simulink model "SensorFusionCompare"  (R2024b)
settings: Solver=FixedStepAuto  StartTime=0.0  StopTime=inf  RelTol=1e-3  EnableMultiTasking=on
values from neighbouring files (symbols this model uses):
  A_kalman = [1 delta_t ... (first row only)    [AttitudePlayground_Vars.m]    (also in ControlSystem_Vars.m)
  acc_sigma = 0.2 * calc_sigma(acc_pp)    [AttitudePlayground_Vars.m]    (also in ControlSystem_Vars.m)
  amfitrack_time = 1    [ControlSystem_Vars.m]
  C_kalman = eye(2)    [AttitudePlayground_Vars.m]    (also in ControlSystem_Vars.m)
  delta_t = 0.01    [AttitudePlayground_Vars.m]    (also in ControlSystem_Vars.m; ParameterIdentification.m = t2 - t1)
  gyro_sigma_3d = [1*gyro_sigma, 1*gyro_sigma, gyro_sigma]    [AttitudePlayground_Vars.m]    (also in ControlSystem_Vars.m)
  inbuilt_reset_time = amfitrack_time + 1    (= 2)    [ControlSystem_Vars.m]
  P_0 = eye(4)    [AttitudePlayground_Vars.m]    (also in ControlSystem_Vars.m)
  q_sigma = 0.001    [AttitudePlayground_Vars.m]    (also in ControlSystem_Vars.m)
  R_kalman = diag([(calc_sigma(0.8))^2, (0.07)^2])    [AttitudePlayground_Vars.m]    (also in ControlSystem_Vars.m)
undefined symbols (not defined in the file or in its folder): Discrete, Time
libraries: simulink_extras x8, dspsigops x2, ctrlSharedLib x1, bbblueSensorLib x1, sharedutil x1, bbblueCommlib x1
settings Model: ExtModeTrigDuration=100  Creator=Henrik  LastModifiedBy=Henrik
settings SolverCC: PositivePriorityOrder=on
settings OptimizationCC: DefaultParameterBehavior=Inlined  EnhancedBackFolding=on  PassReuseOutputArgsAs=Individual arguments  ZeroExternalMemoryAtStartup=off  ZeroInternalMemoryAtStartup=off  MaxStackSize=64  OptimizeBlockOrder=speed  DifferentSizesBufferReuse=on  OptimizationCustomize=off  EfficientTunableParamExpr=on
settings DebuggingCC: ParameterTunabilityLossMsg=error
settings HardwareCC: ProdBitPerPointer=32  ProdBitPerSizeT=32  ProdBitPerPtrDiffT=32  ProdLargestAtomicInteger=Long  ProdLargestAtomicFloat=Double  ProdWordSize=32  ProdHWDeviceType=ARM Compatible->ARM Cortex-A (32-bit)  UseEmbeddedCoderFeatures=off
settings SFSimCC: MATLABDynamicMemAlloc=off
settings RTWCC: Description=Embedded Coder  SystemTargetFile=ert.tlc  HardwareBoard=BeagleBone Blue  TLCOptions="-aInlineSetEventsForThisBaseRateFcn=TLC_FALSE -aSuppressMultiTaskScheduler=TLC_FALSE  -aRateBasedStepFcn=0"  TemplateMakefile=ert_default_tmf  Toolchain=GNU GCC BeagleBone Blue
settings CodeAppCC: ForceParamTrailComments=on  IgnoreCustomStorageClasses=off  OperatorAnnotations=on  SimulinkDataObjDesc=on  SFDataObjDesc=on  InsertBlockDesc=on
settings ERTTargetCC: SupportNonInlinedSFcns=on  SupportVariableSizeSignals=on

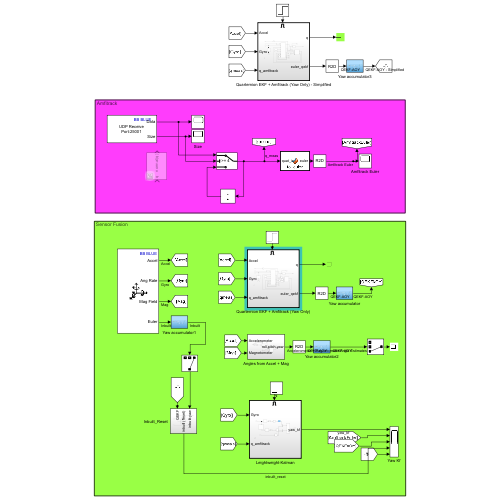
[thumbnail: Simulink's stored preview of the top-level diagram]
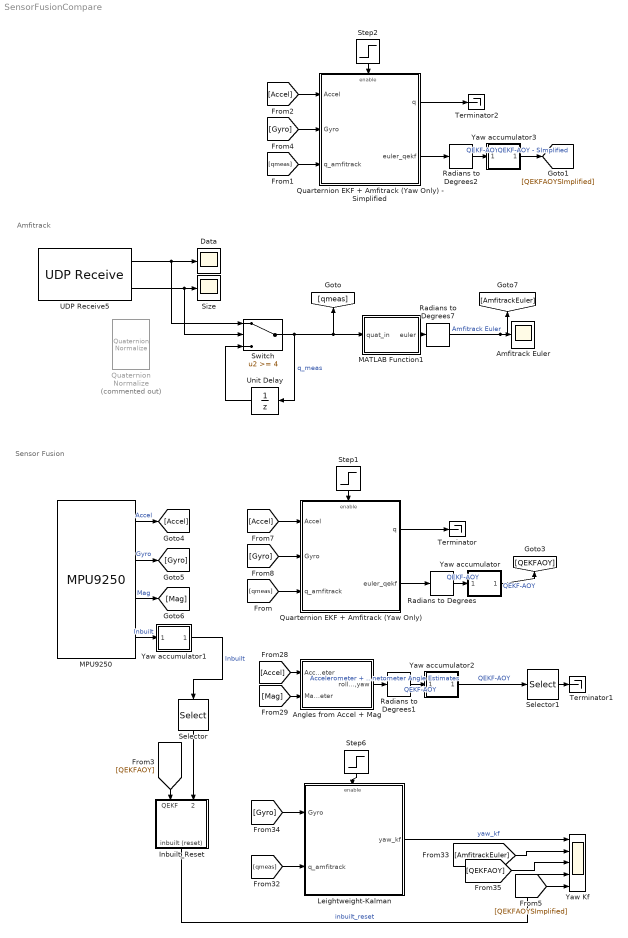
== system SensorFusionCompare ==
  note: Sensor Fusion
  note: Amfitrack
  Amfitrack Euler : Scope
  Angles from Accel + Mag : Subsystem
  Data : Scope
  Inbuilt_Reset : Subsystem
  Leightweight-Kalman : Subsystem
  MATLAB Function1 : MATLAB Function  TreatAsAtomicUnit=on
  MPU9250 : bbblueSensorLib/MPU9250  OperationMode=DMP  Accel=on  AngularRate=on  Ak8963Field=on  EulerAngles=on  Quat=off  AccelRange=2G  Acceldlpf=1  GyroRange=250 dps  Gyrodlpf=1  DmpOdr=200 Hz  SampleTime=delta_t
  Quarternion EKF + Amfitrack (Yaw Only) : Subsystem
  Quarternion EKF + Amfitrack (Yaw Only) - Simplified : Subsystem
  Quaternion Normalize : sharedutil/Quaternion Normalize  Commented=on  aMode=aMode
  Radians to Degrees{,1..2,7} (4 alike) : simulink_extras/Transformations/Radians to Degrees
  Selector : Selector  InputPortWidth=3  IndexOptions=Index vector (dialog)  Indices=[3]  OutputSizes=1
  Selector1 : Selector  InputPortWidth=3  IndexOptions=Index vector (dialog)  Indices=[3]  OutputSizes=1
  Size : Scope
  Step1 : Step  Time=amfitrack_time  SampleTime=delta_t
  Step2 : Step  Time=amfitrack_time  SampleTime=delta_t
  Step6 : Step  Time=amfitrack_time  SampleTime=delta_t
  Switch : Switch  Threshold=4  SaturateOnIntegerOverflow=off  InputSameDT=off
  Terminator : Terminator
  Terminator1 : Terminator
  Terminator2 : Terminator
  UDP Receive5 : bbblueCommlib/UDP Receive  localURL='0.0.0.0'  localPort=25001  remoteURL='0.0.0.0'  remotePort=-1  recvBufferSize=8192  signalDatatype=double  dims=4  isVarSize=off  showBlockingTime=off  blockingTime=0  sampletime=delta_t  blockPlatform=BB BLUE
  Unit Delay : UnitDelay  InitialCondition=[1,0,0,0]'  SampleTime=-1  HasFrameUpgradeWarning=on
  Yaw Kf : Scope  NumInputPorts=5
  Yaw accumulator : Subsystem
  Yaw accumulator1 : Subsystem
  Yaw accumulator2 : Subsystem
  Yaw accumulator3 : Subsystem
  wires:
  MPU9250/1 -> [Accel]  "Accel"
  [Accel] -> Quarternion EKF + Amfitrack (Yaw Only)/1(Accel)
  Radians to Degrees/1 -> Yaw accumulator/1(yaw)  "QEKF-AOY"
  Step1/1 -> Quarternion EKF + Amfitrack (Yaw Only)/Enable
  [Gyro] -> Quarternion EKF + Amfitrack (Yaw Only)/2(Gyro)
  MPU9250/4 -> Yaw accumulator1/1(yaw)  "Inbuilt"
  Angles from Accel + Mag/1(roll,pitch,yaw) -> Radians to Degrees1/1  "Accelerometer + Magnetometer Angle Estimates"
  Quarternion EKF + Amfitrack (Yaw Only)/1(q) -> Terminator/1
  [Accel] -> Angles from Accel + Mag/1(Accelerometer)
  Yaw accumulator2/1(yaw_acc) -> Selector1/1  "QEKF-AOY"
  MPU9250/2 -> [Gyro]  "Gyro"
  Yaw accumulator/1(yaw_acc) -> [QEKFAOY]  "QEKF-AOY"
  Quarternion EKF + Amfitrack (Yaw Only)/2(euler_qekf) -> Radians to Degrees/1
  [qmeas] -> Quarternion EKF + Amfitrack (Yaw Only)/3(q_amfitrack)
  MPU9250/3 -> [Mag]  "Mag"
  Radians to Degrees1/1 -> Yaw accumulator2/1(yaw)  "QEKF-AOY"
  Yaw accumulator1/1(yaw_acc) -> Selector/1  "Inbuilt"
  [Mag] -> Angles from Accel + Mag/2(Magnetometer)
  [AmfitrackEuler] -> Yaw Kf/2
  [Gyro] -> Leightweight-Kalman/1(Gyro)
  Leightweight-Kalman/1(yaw_kf) -> Yaw Kf/1  "yaw_kf"
  [QEKFAOY] -> Yaw Kf/3
  [qmeas] -> Leightweight-Kalman/2(q_amfitrack)
  Step6/1 -> Leightweight-Kalman/Enable
  UDP Receive5/1 -> Switch/1, Data/1
  Switch/1 -> MATLAB Function1/1(quat_in), [qmeas], Unit Delay/1  "q_meas"
  Radians to Degrees7/1 -> Amfitrack Euler/1, [AmfitrackEuler]  "Amfitrack Euler"
  MATLAB Function1/1(euler) -> Radians to Degrees7/1
  Unit Delay/1 -> Switch/3
  UDP Receive5/2 -> Switch/2, Size/1
  [QEKFAOY] -> Inbuilt_Reset/1(QEKF)
  Selector/1 -> Inbuilt_Reset/2(inbuilt-yaw)
  Inbuilt_Reset/1(inbuilt (reset)) -> Yaw Kf/4  "inbuilt_reset"
  Selector1/1 -> Terminator1/1
  [qmeas] -> Quarternion EKF + Amfitrack (Yaw Only) - Simplified/3(q_amfitrack)
  Quarternion EKF + Amfitrack (Yaw Only) - Simplified/2(euler_qekf) -> Radians to Degrees2/1
  Quarternion EKF + Amfitrack (Yaw Only) - Simplified/1(q) -> Terminator2/1
  [Gyro] -> Quarternion EKF + Amfitrack (Yaw Only) - Simplified/2(Gyro)
  Step2/1 -> Quarternion EKF + Amfitrack (Yaw Only) - Simplified/Enable
  Radians to Degrees2/1 -> Yaw accumulator3/1(yaw)  "QEKF-AOY"
  [Accel] -> Quarternion EKF + Amfitrack (Yaw Only) - Simplified/1(Accel)
  Yaw accumulator3/1(yaw_acc) -> [QEKFAOYSImplified]  "QEKF-AOY - SImplified"
  [QEKFAOYSImplified] -> Yaw Kf/5

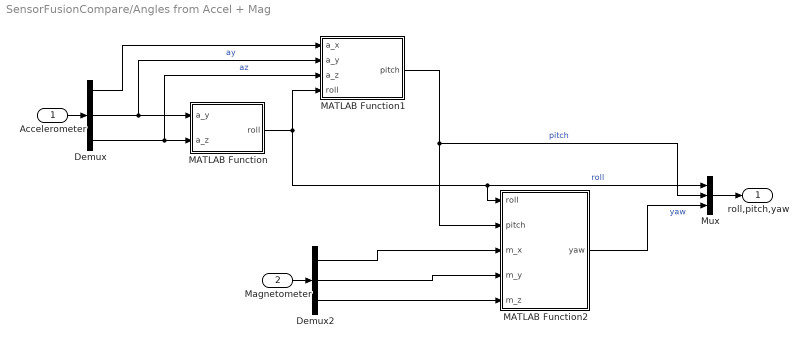
== system SensorFusionCompare/Angles from Accel + Mag ==
  Accelerometer : Inport
  Magnetometer : Inport  Port=2
  Demux : Demux  Outputs=3
  Demux2 : Demux  Outputs=3
  MATLAB Function : MATLAB Function  TreatAsAtomicUnit=on
  MATLAB Function1 : MATLAB Function  TreatAsAtomicUnit=on
  MATLAB Function2 : MATLAB Function  TreatAsAtomicUnit=on
  Mux : Mux  Inputs=3
  roll,pitch,yaw : Outport
  wires:
  Accelerometer/1 -> Demux/1
  Demux/1 -> MATLAB Function1/1(a_x)
  Demux/3 -> MATLAB Function1/3(a_z), MATLAB Function/2(a_z)  "az"
  Demux/2 -> MATLAB Function1/2(a_y), MATLAB Function/1(a_y)  "ay"
  Magnetometer/1 -> Demux2/1
  MATLAB Function/1(roll) -> MATLAB Function1/4(roll), Mux/1, MATLAB Function2/1(roll)  "roll"
  MATLAB Function1/1(pitch) -> Mux/2, MATLAB Function2/2(pitch)  "pitch"
  Demux2/1 -> MATLAB Function2/3(m_x)
  Demux2/2 -> MATLAB Function2/4(m_y)
  Demux2/3 -> MATLAB Function2/5(m_z)
  Mux/1 -> roll,pitch,yaw/1
  MATLAB Function2/1(yaw) -> Mux/3  "yaw"

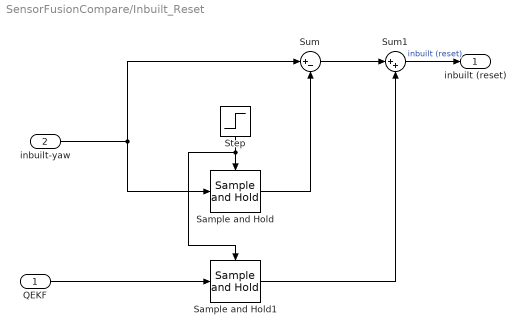
== system SensorFusionCompare/Inbuilt_Reset ==
  QEKF : Inport
  inbuilt-yaw : Inport  Port=2
  Sample and Hold : dspsigops/Sample and Hold  trig=Rising edge  initCond=0  latchinput=off
  Sample and Hold1 : dspsigops/Sample and Hold  trig=Rising edge  initCond=0  latchinput=off
  Step : Step  Time=inbuilt_reset_time  SampleTime=0
  Sum : Sum  Inputs=|+-
  Sum1 : Sum  Inputs=|++
  inbuilt (reset) : Outport
  wires:
  Step/1 -> Sample and Hold1/Trigger, Sample and Hold/Trigger
  Sum/1 -> Sum1/1
  Sample and Hold/1 -> Sum/2
  inbuilt-yaw/1 -> Sum/1, Sample and Hold/1
  Sample and Hold1/1 -> Sum1/2
  Sum1/1 -> inbuilt (reset)/1  "inbuilt (reset)"
  QEKF/1 -> Sample and Hold1/1

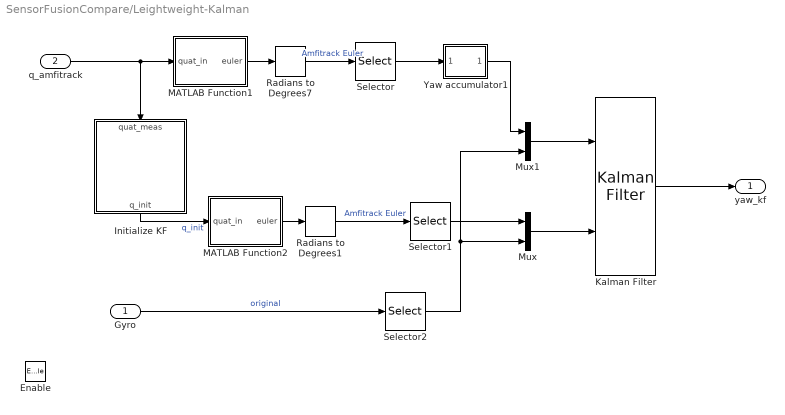
== system SensorFusionCompare/Leightweight-Kalman ==
  Gyro : Inport
  q_amfitrack : Inport  Port=2
  Enable : EnablePort
  Initialize KF : MATLAB Function  TreatAsAtomicUnit=on
  Kalman Filter : ctrlSharedLib/Kalman Filter  TimeDomain=Discrete-Time  UseCurrentEstimator=on  ModelSource=Individual A, B, C, D matrices  ModelSourceVariable=ss(0.95,1,1,0,1)  A=A_kalman  B=1  C=C_kalman  D=0  NumberOfStates=1  NumberOfInputs=1  NumberOfOutputs=1  InitialEstimateSource=Input port  X0=0  P0=10  UseK=off  UseGH=off  NumberOfProcessNoiseInputs=1  G=1  TimeInvariantG=on  H=0  TimeInvariantH=on  Q=Q_kalman  TimeInvariantQ=on  R=R_kalman  TimeInvariantR=on  N=0  TimeInvariantN=on  AddInputPort=off  AddEnablePort=off  OutputEstimatedY=off  OutputP=off  Ts=-1
  MATLAB Function1 : MATLAB Function  TreatAsAtomicUnit=on
  MATLAB Function2 : MATLAB Function  TreatAsAtomicUnit=on
  Mux : Mux  Inputs=2
  Mux1 : Mux  Inputs=2
  Radians to Degrees1 : simulink_extras/Transformations/Radians to Degrees
  Radians to Degrees7 : simulink_extras/Transformations/Radians to Degrees
  Selector : Selector  InputPortWidth=3  IndexOptions=Index vector (dialog)  Indices=[3]  OutputSizes=1
  Selector1 : Selector  InputPortWidth=3  IndexOptions=Index vector (dialog)  Indices=[3]  OutputSizes=1
  Selector2 : Selector  InputPortWidth=3  IndexOptions=Index vector (dialog)  Indices=[3]  OutputSizes=1
  Yaw accumulator1 : Subsystem
  yaw_kf : Outport
  wires:
  Gyro/1 -> Selector2/1  "original"
  q_amfitrack/1 -> MATLAB Function1/1(quat_in), Initialize KF/1(quat_meas)
  Initialize KF/1(q_init) -> MATLAB Function2/1(quat_in)  "q_init"
  Radians to Degrees7/1 -> Selector/1  "Amfitrack Euler"
  MATLAB Function1/1(euler) -> Radians to Degrees7/1
  MATLAB Function2/1(euler) -> Radians to Degrees1/1
  Radians to Degrees1/1 -> Selector1/1  "Amfitrack Euler"
  Selector1/1 -> Mux/1
  Mux/1 -> Kalman Filter/2
  Kalman Filter/1 -> yaw_kf/1
  Selector/1 -> Yaw accumulator1/1(yaw)
  Mux1/1 -> Kalman Filter/1
  Yaw accumulator1/1(yaw_acc) -> Mux1/1
  Selector2/1 -> Mux1/2, Mux/2

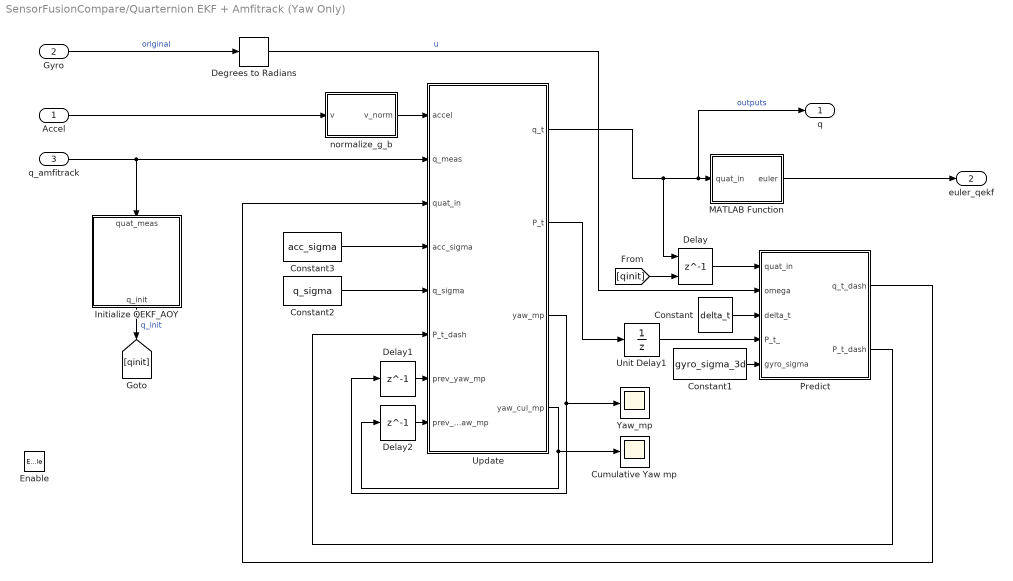
== system SensorFusionCompare/Quarternion EKF + Amfitrack (Yaw Only) ==
  Accel : Inport
  Gyro : Inport  Port=2
  q_amfitrack : Inport  Port=3
  Enable : EnablePort
  Constant : Constant  Value=delta_t
  Constant1 : Constant  Value=gyro_sigma_3d
  Constant2 : Constant  Value=q_sigma
  Constant3 : Constant  Value=acc_sigma
  Cumulative Yaw mp : Scope
  Degrees to Radians : simulink_extras/Transformations/Degrees to Radians
  Delay : Delay  DelayLength=1  InitialConditionSource=Input port  InitialCondition=[1,0,0,0]  SampleTime=delta_t
      settings: InputPortMap=u0,p4
  Delay1 : Delay  DelayLength=1  InitialCondition=[0,0]  SampleTime=delta_t
  Delay2 : Delay  DelayLength=1  InitialCondition=[0,0]  SampleTime=delta_t
  Initialize QEKF_AOY : MATLAB Function  TreatAsAtomicUnit=on
  MATLAB Function : MATLAB Function  TreatAsAtomicUnit=on
  Predict : MATLAB Function  TreatAsAtomicUnit=on
  Unit Delay1 : UnitDelay  InitialCondition=P_0  SampleTime=delta_t  HasFrameUpgradeWarning=on
  Update : MATLAB Function  TreatAsAtomicUnit=on  SystemSampleTime=delta_t
  Yaw_mp : Scope
  normalize_g_b : MATLAB Function  TreatAsAtomicUnit=on
  q : Outport
  euler_qekf : Outport  Port=2
  wires:
  Update/1(q_t) -> Delay/1, q/1, MATLAB Function/1(quat_in)  "outputs"
  Accel/1 -> normalize_g_b/1(v)
  Constant/1 -> Predict/3(delta_t)
  Unit Delay1/1 -> Predict/4(P_t_)
  Update/2(P_t) -> Unit Delay1/1
  Predict/1(q_t_dash) -> Update/3(quat_in)
  normalize_g_b/1(v_norm) -> Update/1(accel)
  Constant3/1 -> Update/4(acc_sigma)
  Delay/1 -> Predict/1(quat_in)
  Predict/2(P_t_dash) -> Update/6(P_t_dash)
  MATLAB Function/1(euler) -> euler_qekf/1
  Degrees to Radians/1 -> Predict/2(omega)  "u"
  Gyro/1 -> Degrees to Radians/1  "original"
  Constant1/1 -> Predict/5(gyro_sigma)
  q_amfitrack/1 -> Update/2(q_meas), Initialize QEKF_AOY/1(quat_meas)
  Constant2/1 -> Update/5(q_sigma)
  Delay1/1 -> Update/7(prev_yaw_mp)
  Delay2/1 -> Update/8(prev_cul_yaw_mp)
  Update/3(yaw_mp) -> Delay1/1, Yaw_mp/1
  Update/4(yaw_cul_mp) -> Delay2/1, Cumulative Yaw mp/1
  Initialize QEKF_AOY/1(q_init) -> [qinit]  "q_init"
  [qinit] -> Delay/2

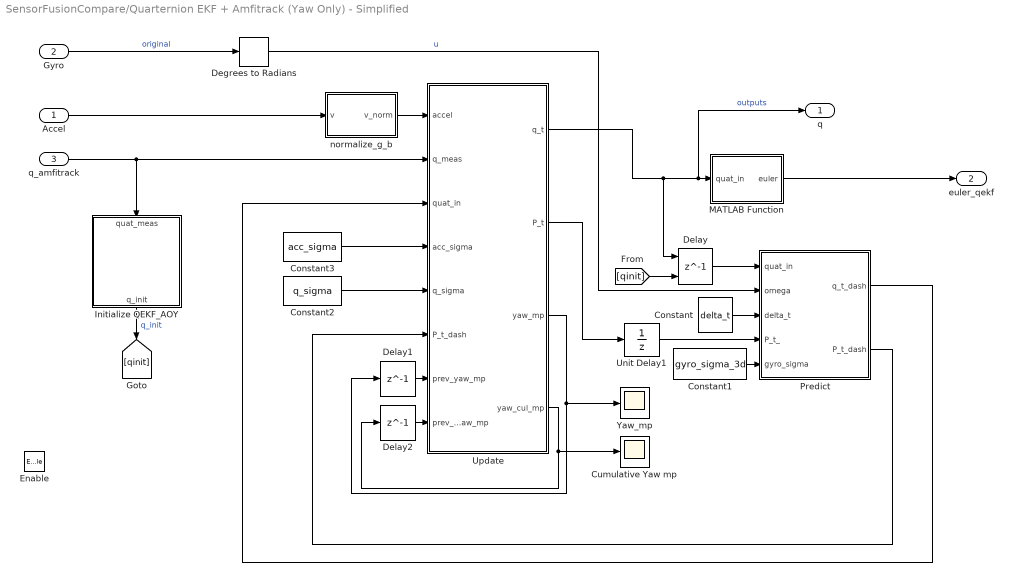
== system SensorFusionCompare/Quarternion EKF + Amfitrack (Yaw Only) - Simplified ==
  Accel : Inport
  Gyro : Inport  Port=2
  q_amfitrack : Inport  Port=3
  Enable : EnablePort
  Constant : Constant  Value=delta_t
  Constant1 : Constant  Value=gyro_sigma_3d
  Constant2 : Constant  Value=q_sigma
  Constant3 : Constant  Value=acc_sigma
  Cumulative Yaw mp : Scope
  Degrees to Radians : simulink_extras/Transformations/Degrees to Radians
  Delay : Delay  DelayLength=1  InitialConditionSource=Input port  InitialCondition=[1,0,0,0]  SampleTime=delta_t
      settings: InputPortMap=u0,p4
  Delay1 : Delay  DelayLength=1  InitialCondition=[0,0]  SampleTime=delta_t
  Delay2 : Delay  DelayLength=1  InitialCondition=[0,0]  SampleTime=delta_t
  Initialize QEKF_AOY : MATLAB Function  TreatAsAtomicUnit=on
  MATLAB Function : MATLAB Function  TreatAsAtomicUnit=on
  Predict : MATLAB Function  TreatAsAtomicUnit=on
  Unit Delay1 : UnitDelay  InitialCondition=P_0  SampleTime=delta_t  HasFrameUpgradeWarning=on
  Update : MATLAB Function  TreatAsAtomicUnit=on  SystemSampleTime=delta_t
  Yaw_mp : Scope
  normalize_g_b : MATLAB Function  TreatAsAtomicUnit=on
  q : Outport
  euler_qekf : Outport  Port=2
  wires:
  [qinit] -> Delay/2
  Initialize QEKF_AOY/1(q_init) -> [qinit]  "q_init"
  Update/4(yaw_cul_mp) -> Cumulative Yaw mp/1, Delay2/1
  Update/3(yaw_mp) -> Yaw_mp/1, Delay1/1
  Delay2/1 -> Update/8(prev_cul_yaw_mp)
  Delay1/1 -> Update/7(prev_yaw_mp)
  Constant2/1 -> Update/5(q_sigma)
  q_amfitrack/1 -> Initialize QEKF_AOY/1(quat_meas), Update/2(q_meas)
  Constant1/1 -> Predict/5(gyro_sigma)
  Gyro/1 -> Degrees to Radians/1  "original"
  Degrees to Radians/1 -> Predict/2(omega)  "u"
  MATLAB Function/1(euler) -> euler_qekf/1
  Predict/2(P_t_dash) -> Update/6(P_t_dash)
  Delay/1 -> Predict/1(quat_in)
  Constant3/1 -> Update/4(acc_sigma)
  normalize_g_b/1(v_norm) -> Update/1(accel)
  Predict/1(q_t_dash) -> Update/3(quat_in)
  Update/2(P_t) -> Unit Delay1/1
  Unit Delay1/1 -> Predict/4(P_t_)
  Constant/1 -> Predict/3(delta_t)
  Accel/1 -> normalize_g_b/1(v)
  Update/1(q_t) -> MATLAB Function/1(quat_in), q/1, Delay/1  "outputs"

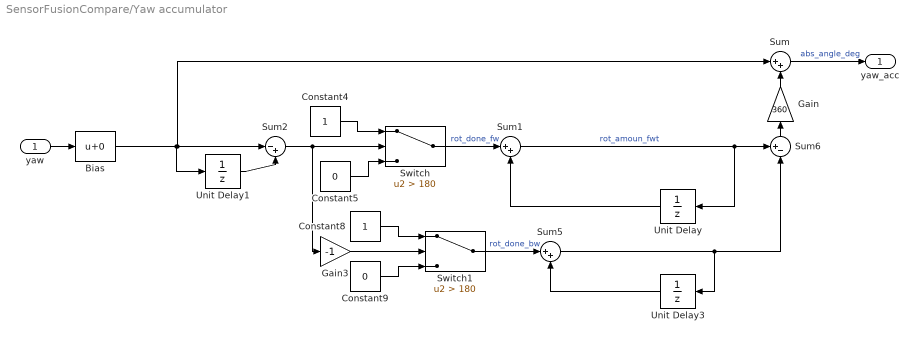
== system SensorFusionCompare/Yaw accumulator ==
  yaw : Inport
  Bias : Bias  SaturateOnIntegerOverflow=off
  Constant4 : Constant
  Constant5 : Constant  Value=0
  Constant8 : Constant
  Constant9 : Constant  Value=0
  Gain : Gain  Gain=360
  Gain3 : Gain  Gain=-1
  Sum : Sum  Inputs=|++
  Sum1 : Sum  Inputs=|++
  Sum2 : Sum  Inputs=|-+
  Sum5 : Sum  Inputs=|++
  Sum6 : Sum  Inputs=+-|
  Switch : Switch  Criteria=u2 > Threshold  Threshold=180  SaturateOnIntegerOverflow=off  InputSameDT=off
  Switch1 : Switch  Criteria=u2 > Threshold  Threshold=180  SaturateOnIntegerOverflow=off  InputSameDT=off
  Unit Delay : UnitDelay  SampleTime=-1  HasFrameUpgradeWarning=on
  Unit Delay1 : UnitDelay  SampleTime=-1  HasFrameUpgradeWarning=on
  Unit Delay3 : UnitDelay  SampleTime=-1  HasFrameUpgradeWarning=on
  yaw_acc : Outport
  wires:
  Sum1/1 -> Unit Delay/1, Sum6/1  "rot_amoun_fwt"
  Constant5/1 -> Switch/3
  Constant8/1 -> Switch1/1
  Sum5/1 -> Unit Delay3/1, Sum6/2
  Sum6/1 -> Gain/1
  Unit Delay/1 -> Sum1/2
  Constant4/1 -> Switch/1
  yaw/1 -> Bias/1
  Unit Delay3/1 -> Sum5/2
  Switch/1 -> Sum1/1  "rot_done_fw"
  Sum2/1 -> Gain3/1, Switch/2
  Gain3/1 -> Switch1/2
  Unit Delay1/1 -> Sum2/2
  Sum/1 -> yaw_acc/1  "abs_angle_deg"
  Switch1/1 -> Sum5/1  "rot_done_bw"
  Constant9/1 -> Switch1/3
  Gain/1 -> Sum/2
  Bias/1 -> Unit Delay1/1, Sum/1, Sum2/1

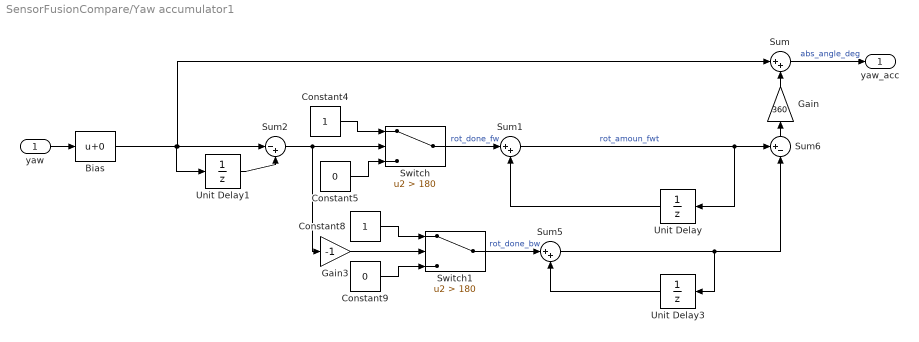
== system SensorFusionCompare/Yaw accumulator1 ==
  yaw : Inport
  Bias : Bias  SaturateOnIntegerOverflow=off
  Constant4 : Constant
  Constant5 : Constant  Value=0
  Constant8 : Constant
  Constant9 : Constant  Value=0
  Gain : Gain  Gain=360
  Gain3 : Gain  Gain=-1
  Sum : Sum  Inputs=|++
  Sum1 : Sum  Inputs=|++
  Sum2 : Sum  Inputs=|-+
  Sum5 : Sum  Inputs=|++
  Sum6 : Sum  Inputs=+-|
  Switch : Switch  Criteria=u2 > Threshold  Threshold=180  SaturateOnIntegerOverflow=off  InputSameDT=off
  Switch1 : Switch  Criteria=u2 > Threshold  Threshold=180  SaturateOnIntegerOverflow=off  InputSameDT=off
  Unit Delay : UnitDelay  SampleTime=-1  HasFrameUpgradeWarning=on
  Unit Delay1 : UnitDelay  SampleTime=-1  HasFrameUpgradeWarning=on
  Unit Delay3 : UnitDelay  SampleTime=-1  HasFrameUpgradeWarning=on
  yaw_acc : Outport
  wires:
  Sum1/1 -> Unit Delay/1, Sum6/1  "rot_amoun_fwt"
  Constant5/1 -> Switch/3
  Constant8/1 -> Switch1/1
  Sum5/1 -> Unit Delay3/1, Sum6/2
  Sum6/1 -> Gain/1
  Unit Delay/1 -> Sum1/2
  Constant4/1 -> Switch/1
  yaw/1 -> Bias/1
  Unit Delay3/1 -> Sum5/2
  Switch/1 -> Sum1/1  "rot_done_fw"
  Sum2/1 -> Gain3/1, Switch/2
  Gain3/1 -> Switch1/2
  Unit Delay1/1 -> Sum2/2
  Sum/1 -> yaw_acc/1  "abs_angle_deg"
  Switch1/1 -> Sum5/1  "rot_done_bw"
  Constant9/1 -> Switch1/3
  Gain/1 -> Sum/2
  Bias/1 -> Unit Delay1/1, Sum/1, Sum2/1

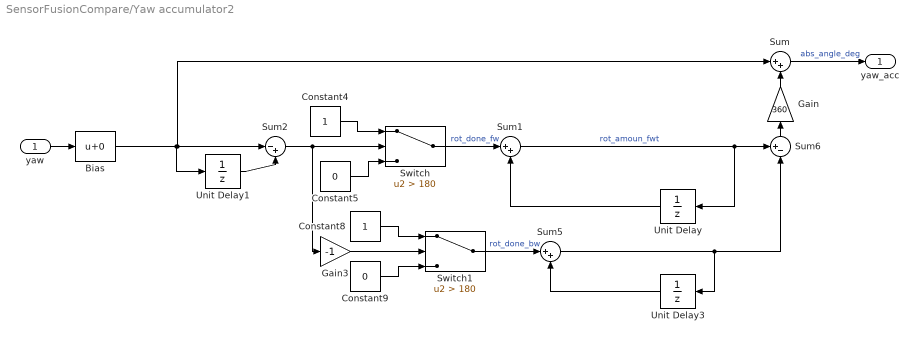
== system SensorFusionCompare/Yaw accumulator2 ==
  yaw : Inport
  Bias : Bias  SaturateOnIntegerOverflow=off
  Constant4 : Constant
  Constant5 : Constant  Value=0
  Constant8 : Constant
  Constant9 : Constant  Value=0
  Gain : Gain  Gain=360
  Gain3 : Gain  Gain=-1
  Sum : Sum  Inputs=|++
  Sum1 : Sum  Inputs=|++
  Sum2 : Sum  Inputs=|-+
  Sum5 : Sum  Inputs=|++
  Sum6 : Sum  Inputs=+-|
  Switch : Switch  Criteria=u2 > Threshold  Threshold=180  SaturateOnIntegerOverflow=off  InputSameDT=off
  Switch1 : Switch  Criteria=u2 > Threshold  Threshold=180  SaturateOnIntegerOverflow=off  InputSameDT=off
  Unit Delay : UnitDelay  SampleTime=-1  HasFrameUpgradeWarning=on
  Unit Delay1 : UnitDelay  SampleTime=-1  HasFrameUpgradeWarning=on
  Unit Delay3 : UnitDelay  SampleTime=-1  HasFrameUpgradeWarning=on
  yaw_acc : Outport
  wires:
  Bias/1 -> Sum2/1, Sum/1, Unit Delay1/1
  Gain/1 -> Sum/2
  Constant9/1 -> Switch1/3
  Switch1/1 -> Sum5/1  "rot_done_bw"
  Sum/1 -> yaw_acc/1  "abs_angle_deg"
  Unit Delay1/1 -> Sum2/2
  Gain3/1 -> Switch1/2
  Sum2/1 -> Switch/2, Gain3/1
  Switch/1 -> Sum1/1  "rot_done_fw"
  Unit Delay3/1 -> Sum5/2
  yaw/1 -> Bias/1
  Constant4/1 -> Switch/1
  Unit Delay/1 -> Sum1/2
  Sum6/1 -> Gain/1
  Sum5/1 -> Sum6/2, Unit Delay3/1
  Constant8/1 -> Switch1/1
  Constant5/1 -> Switch/3
  Sum1/1 -> Sum6/1, Unit Delay/1  "rot_amoun_fwt"

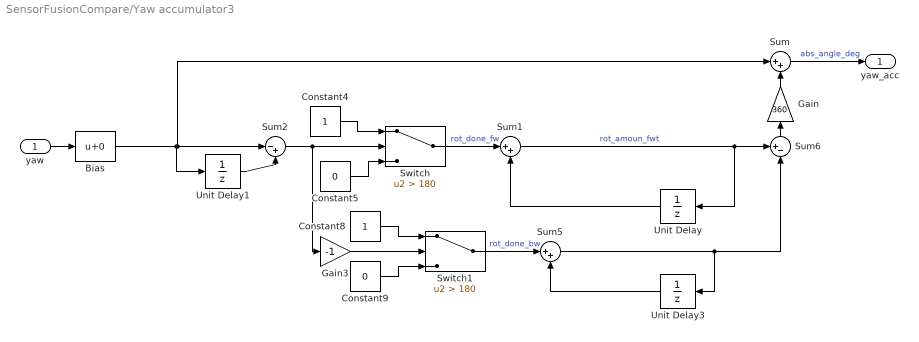
== system SensorFusionCompare/Yaw accumulator3 ==
  yaw : Inport
  Bias : Bias  SaturateOnIntegerOverflow=off
  Constant4 : Constant
  Constant5 : Constant  Value=0
  Constant8 : Constant
  Constant9 : Constant  Value=0
  Gain : Gain  Gain=360
  Gain3 : Gain  Gain=-1
  Sum : Sum  Inputs=|++
  Sum1 : Sum  Inputs=|++
  Sum2 : Sum  Inputs=|-+
  Sum5 : Sum  Inputs=|++
  Sum6 : Sum  Inputs=+-|
  Switch : Switch  Criteria=u2 > Threshold  Threshold=180  SaturateOnIntegerOverflow=off  InputSameDT=off
  Switch1 : Switch  Criteria=u2 > Threshold  Threshold=180  SaturateOnIntegerOverflow=off  InputSameDT=off
  Unit Delay : UnitDelay  SampleTime=-1  HasFrameUpgradeWarning=on
  Unit Delay1 : UnitDelay  SampleTime=-1  HasFrameUpgradeWarning=on
  Unit Delay3 : UnitDelay  SampleTime=-1  HasFrameUpgradeWarning=on
  yaw_acc : Outport
  wires:
  Bias/1 -> Sum2/1, Sum/1, Unit Delay1/1
  Gain/1 -> Sum/2
  Constant9/1 -> Switch1/3
  Switch1/1 -> Sum5/1  "rot_done_bw"
  Sum/1 -> yaw_acc/1  "abs_angle_deg"
  Unit Delay1/1 -> Sum2/2
  Gain3/1 -> Switch1/2
  Sum2/1 -> Switch/2, Gain3/1
  Switch/1 -> Sum1/1  "rot_done_fw"
  Unit Delay3/1 -> Sum5/2
  yaw/1 -> Bias/1
  Constant4/1 -> Switch/1
  Unit Delay/1 -> Sum1/2
  Sum6/1 -> Gain/1
  Sum5/1 -> Sum6/2, Unit Delay3/1
  Constant8/1 -> Switch1/1
  Constant5/1 -> Switch/3
  Sum1/1 -> Sum6/1, Unit Delay/1  "rot_amoun_fwt"

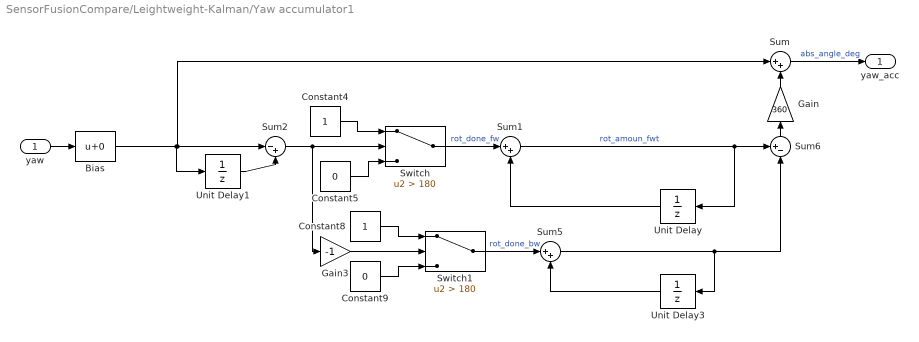
== system SensorFusionCompare/Leightweight-Kalman/Yaw accumulator1 ==
  yaw : Inport
  Bias : Bias  SaturateOnIntegerOverflow=off
  Constant4 : Constant
  Constant5 : Constant  Value=0
  Constant8 : Constant
  Constant9 : Constant  Value=0
  Gain : Gain  Gain=360
  Gain3 : Gain  Gain=-1
  Sum : Sum  Inputs=|++
  Sum1 : Sum  Inputs=|++
  Sum2 : Sum  Inputs=|-+
  Sum5 : Sum  Inputs=|++
  Sum6 : Sum  Inputs=+-|
  Switch : Switch  Criteria=u2 > Threshold  Threshold=180  SaturateOnIntegerOverflow=off  InputSameDT=off
  Switch1 : Switch  Criteria=u2 > Threshold  Threshold=180  SaturateOnIntegerOverflow=off  InputSameDT=off
  Unit Delay : UnitDelay  SampleTime=-1  HasFrameUpgradeWarning=on
  Unit Delay1 : UnitDelay  SampleTime=-1  HasFrameUpgradeWarning=on
  Unit Delay3 : UnitDelay  SampleTime=-1  HasFrameUpgradeWarning=on
  yaw_acc : Outport
  wires:
  Sum1/1 -> Unit Delay/1, Sum6/1  "rot_amoun_fwt"
  Constant5/1 -> Switch/3
  Constant8/1 -> Switch1/1
  Sum5/1 -> Unit Delay3/1, Sum6/2
  Sum6/1 -> Gain/1
  Unit Delay/1 -> Sum1/2
  Constant4/1 -> Switch/1
  yaw/1 -> Bias/1
  Unit Delay3/1 -> Sum5/2
  Switch/1 -> Sum1/1  "rot_done_fw"
  Sum2/1 -> Gain3/1, Switch/2
  Gain3/1 -> Switch1/2
  Unit Delay1/1 -> Sum2/2
  Sum/1 -> yaw_acc/1  "abs_angle_deg"
  Switch1/1 -> Sum5/1  "rot_done_bw"
  Constant9/1 -> Switch1/3
  Gain/1 -> Sum/2
  Bias/1 -> Unit Delay1/1, Sum/1, Sum2/1

== matlab function SensorFusionCompare/Leightweight-Kalman/Initialize KF ==
  data: quat_meas input; q_init output
function q_init = calc_init_q(quat_meas)

q0 = quat_meas(1);
q1 = quat_meas(2);
q2 = quat_meas(3);
q3 = quat_meas(4);


yaw_init_rad = atan2((2 * (q0*q3 + q1*q2)),(1 - 2*(q2^2 + q3^2)));
q_init = [cos(yaw_init_rad/2), 0, 0, sin(yaw_init_rad/2)];

== matlab function SensorFusionCompare/Leightweight-Kalman/MATLAB Function1 ==
  data: quat_in input; euler output
function euler = to_euler(quat_in)

q0 = quat_in(1);
q1 = quat_in(2);
q2 = quat_in(3);
q3 = quat_in(4);

roll = atan((2 * (q0*q1 + q2*q3))/(1 - 2*(q1^2 + q2^2)));
pitch = asin(2 * (q0*q2 - q1*q3));
yaw = atan2((2 * (q0*q3 + q1*q2)),(1 - 2*(q2^2 + q3^2)));

euler = [roll; pitch; yaw];

== matlab function SensorFusionCompare/Leightweight-Kalman/MATLAB Function2 ==
  data: quat_in input; euler output
function euler = to_euler(quat_in)

q0 = quat_in(1);
q1 = quat_in(2);
q2 = quat_in(3);
q3 = quat_in(4);

roll = atan((2 * (q0*q1 + q2*q3))/(1 - 2*(q1^2 + q2^2)));
pitch = asin(2 * (q0*q2 - q1*q3));
yaw = atan2((2 * (q0*q3 + q1*q2)),(1 - 2*(q2^2 + q3^2)));

euler = [roll; pitch; yaw];

== matlab function SensorFusionCompare/MATLAB Function1 ==
  data: quat_in input; euler output
function euler = to_euler(quat_in)

q0 = quat_in(1);
q1 = quat_in(2);
q2 = quat_in(3);
q3 = quat_in(4);

roll = atan((2 * (q0*q1 + q2*q3))/(1 - 2*(q1^2 + q2^2)));
pitch = asin(2 * (q0*q2 - q1*q3));
yaw = atan2((2 * (q0*q3 + q1*q2)),(1 - 2*(q2^2 + q3^2)));

euler = [roll; pitch; yaw];

== matlab function SensorFusionCompare/Quarternion EKF + Amfitrack (Yaw Only)/MATLAB Function ==
  data: quat_in input; euler output
function euler = to_euler(quat_in)

q0 = quat_in(1);
q1 = quat_in(2);
q2 = quat_in(3);
q3 = quat_in(4);

roll = atan((2 * (q0*q1 + q2*q3))/(1 - 2*(q1^2 + q2^2)));
pitch = asin(2 * (q0*q2 - q1*q3));
yaw = atan2((2 * (q0*q3 + q1*q2)),(1 - 2*(q2^2 + q3^2)));

euler = [roll; pitch; yaw];

== matlab function SensorFusionCompare/Quarternion EKF + Amfitrack (Yaw Only)/Predict ==
  data: quat_in input; q_t_dash output; omega input; delta_t input; P_t_dash output; P_t_ input; gyro_sigma input
function [q_t_dash, P_t_dash] = Predict(quat_in, omega, delta_t, P_t_, gyro_sigma)

q0 = quat_in(1);
q1 = quat_in(2);
q2 = quat_in(3);
q3 = quat_in(4);

omega_x = omega(1);
omega_y = omega(2);
omega_z = omega(3);

R_gyro = [gyro_sigma(1)^2 0 0;
          0 gyro_sigma(2)^2 0;
          0 0 gyro_sigma(3)^2;];

q0_out = q0 + delta_t/2 * (-omega_x * q1 - omega_y * q2 - omega_z * q3);
q1_out = q1 + delta_t/2 * ( omega_x * q0 - omega_y * q3 + omega_z * q2);
q2_out = q2 + delta_t/2 * ( omega_x * q3 + omega_y * q0 - omega_z * q1);
q3_out = q3 + delta_t/2 * (-omega_x * q2 + omega_y * q1 + omega_z * q0);

q_t_dash = quatnormalize([q0_out, q1_out, q2_out, q3_out]);

dt2 = delta_t/2;

F = [1  -dt2*omega_x -dt2*omega_y -dt2*omega_z;
    dt2*omega_x    1  dt2*omega_z  dt2*omega_y;
    dt2*omega_y   -dt2*omega_z   1 dt2*omega_x;
    dt2*omega_z    dt2*omega_y -dt2*omega_x  1;
    ];


W = dt2 * [-q1 -q2 -q3;
            q0 -q3  q2;
            q3  q0 -q1;
            -q2 q1  q0]; 

Q_t =  W* R_gyro * W';

P_t_dash = F * P_t_ * F' + Q_t;

== matlab function SensorFusionCompare/Quarternion EKF + Amfitrack (Yaw Only)/Update ==
  data: accel input; q_meas input; q_t output; quat_in input; acc_sigma input; q_sigma input; P_t output; P_t_dash input; prev_yaw_mp input; prev_cul_yaw_mp input; yaw_mp output; yaw_cul_mp output
function [q_t, P_t, yaw_mp, yaw_cul_mp]   = Update(accel, q_meas, quat_in, acc_sigma, q_sigma, P_t_dash, prev_yaw_mp, prev_cul_yaw_mp)

%% Unbox function inputs
q0 = quat_in(1);
q1 = quat_in(2);
q2 = quat_in(3);
q3 = quat_in(4);

q_t_dash = [q0; q1; q2; q3];

yaw_meas_prev = prev_yaw_mp(1);
yaw_meas_cul_prev = prev_cul_yaw_mp(1);
yaw_pred_prev = prev_yaw_mp(2);
yaw_pred_cul_prev = prev_cul_yaw_mp(2);

yaw_meas = atan2((2 * (q_meas(1)*q_meas(4) + q_meas(2)*q_meas(3))),(1 - 2*(q_meas(3)^2 + q_meas(4)^2)));
yaw_pred = atan2((2 * (q0*q3 + q1*q2)),(1 - 2*(q2^2 + q3^2)));

%% Accumulate measured & predicted Yaw Angles
% Determine Change in measured and predicted Yaw angle
delta_yaw_meas = yaw_meas - yaw_meas_prev;
delta_yaw_pred = yaw_pred - yaw_pred_prev;

if delta_yaw_meas > pi
    delta_yaw_meas = delta_yaw_meas - 2*pi;
elseif delta_yaw_meas < -pi
    delta_yaw_meas = delta_yaw_meas + 2*pi;
end

yaw_meas_cul = yaw_meas_cul_prev + delta_yaw_meas;

if delta_yaw_pred > pi
    delta_yaw_pred = delta_yaw_pred - 2*pi;
elseif delta_yaw_pred < -pi
    delta_yaw_pred = delta_yaw_pred + 2*pi;
end

yaw_pred_cul = yaw_pred_cul_prev + delta_yaw_pred;

% Send them to the delay blocks for use in next update step
yaw_mp = [yaw_meas,yaw_pred];
yaw_cul_mp = [yaw_meas_cul, yaw_pred_cul];


%% Update State Estimation

% Construct measurement vector using accumulated yaw angles
z_t = [accel(1);
       accel(2);
       accel(3);
       yaw_meas_cul;
       ];

gx = 0;
gy = 0;
gz = 1;

R = [acc_sigma^2 * eye(3) zeros(3,1);
    zeros(1,3)     q_sigma^2 * eye(1)];

% Measurement Model
h = [
    2*(gx * (1/2 - q2^2 - q3^2) + gy * (q0*q3 + q1*q2) + gz * (q1*q3 - q0*q2));
    2*(gx * (q1*q2 - q0*q3) + gy * (1/2 - q1^2 - q3^2) + gz * (q0*q1 + q2*q3));
    2*(gx * (q0*q2 + q1*q3) + gy * (q2*q3 - q0*q1) + gz * (1/2 - q1^2 - q2^2));
                                    yaw_pred_cul                           ;
                                    
];

% Jacobian of Measurement Model
H = 2 * [
    gx*q0 + gy*q3 - gz*q2,  gx*q1 + gy*q2 + gz*q3, -gx*q2 + gy*q1 - gz*q0, -gx*q3 + gy*q0 + gz*q1;
   -gx*q3 + gy*q0 + gz*q1,  gx*q2 - gy*q1 + gz*q0,  gx*q1 + gy*q2 + gz*q3, -gx*q0 - gy*q3 + gz*q2;
    gx*q2 - gy*q1 + gz*q0,  gx*q3 - gy*q0 - gz*q1,  gx*q0 + gy*q3 - gz*q2,  gx*q1 + gy*q2 + gz*q3;
                                            
    0.5*[-(2*q3*(2*q2^2 + 2*q3^2 - 1))/((2*q2^2 + 2*q3^2 - 1)^2 + (2*q0*q3 + 2*q1*q2)^2), -(2*q2*(2*q2^2 + 2*q3^2 - 1))/((2*q2^2 + 2*q3^2 - 1)^2 + (2*q0*q3 + 2*q1*q2)^2), -(((2*q1)/(2*q2^2 + 2*q3^2 - 1) - (4*q2*(2*q0*q3 + 2*q1*q2))/(2*q2^2 + 2*q3^2 - 1)^2)*(2*q2^2 + 2*q3^2 - 1)^2)/((2*q2^2 + 2*q3^2 - 1)^2 + (2*q0*q3 + 2*q1*q2)^2), -(((2*q0)/(2*q2^2 + 2*q3^2 - 1) - (4*q3*(2*q0*q3 + 2*q1*q2))/(2*q2^2 + 2*q3^2 - 1)^2)*(2*q2^2 + 2*q3^2 - 1)^2)/((2*q2^2 + 2*q3^2 - 1)^2 + (2*q0*q3 + 2*q1*q2)^2)]
];

v_t = z_t - h;

S_t = H * P_t_dash * transpose(H) + R;
K_t = P_t_dash * transpose(H) * inv(S_t);

q_t = quatnormalize(transpose(q_t_dash + K_t*v_t));

P_t = (eye(4) - K_t*H) * P_t_dash;

== matlab function SensorFusionCompare/Quarternion EKF + Amfitrack (Yaw Only)/normalize_g_b ==
  data: v input; v_norm output
function v_norm = normalize_vec(v)

v_norm = v / norm(v);

== matlab function SensorFusionCompare/Quarternion EKF + Amfitrack (Yaw Only)/Initialize QEKF_AOY ==
  data: quat_meas input; q_init output
function q_init = calc_init_q(quat_meas)

q0 = quat_meas(1);
q1 = quat_meas(2);
q2 = quat_meas(3);
q3 = quat_meas(4);


yaw_init_rad = atan2((2 * (q0*q3 + q1*q2)),(1 - 2*(q2^2 + q3^2)));
q_init = [cos(yaw_init_rad/2), 0, 0, sin(yaw_init_rad/2)];

== matlab function SensorFusionCompare/Angles from Accel + Mag/MATLAB Function ==
  data: a_y input; roll output; a_z input
function roll = calc_roll(a_y, a_z)

roll = atan(a_y / a_z);

== matlab function SensorFusionCompare/Quarternion EKF + Amfitrack (Yaw Only) - Simplified/Initialize QEKF_AOY ==
  data: quat_meas input; q_init output
function q_init = calc_init_q(quat_meas)

q0 = quat_meas(1);
q1 = quat_meas(2);
q2 = quat_meas(3);
q3 = quat_meas(4);


yaw_init_rad = atan2((2 * (q0*q3 + q1*q2)),(1 - 2*(q2^2 + q3^2)));
q_init = [cos(yaw_init_rad/2), 0, 0, sin(yaw_init_rad/2)];

== matlab function SensorFusionCompare/Angles from Accel + Mag/MATLAB Function1 ==
  data: a_x input; a_y input; pitch output; a_z input; roll input
function pitch = calc_pitch(a_x, a_y, a_z, roll)

pitch = atan(-a_x / (a_y * sin(roll) + a_z * cos(roll)));

== matlab function SensorFusionCompare/Angles from Accel + Mag/MATLAB Function2 ==
  data: roll input; pitch input; m_x input; yaw output; m_y input; m_z input
function yaw = calc_yaw(roll, pitch, m_x, m_y, m_z)
    % Adjust for roll
    m_x2 = m_x * cos(pitch) + m_z * sin(pitch);
    m_y2 = m_x * sin(roll) * sin(pitch) + m_y * cos(roll) - m_z * sin(roll) * cos(pitch);
    % Calculate yaw
    yaw = atan2(-m_y2, m_x2);



%function yaw = calc_yaw(a_x, pitch, roll, m_x, m_y, m_z)

%m_y2 = m_z * sin(roll) - m_y * cos(roll);
%m_z2 = m_y * sin(roll) - m_z * cos(roll);
%m_x2 = m_x * cos(pitch) + m_z2 * sin(pitch);
%yaw = atan(m_y2/m_x2);

%yaw = atan(-a_x / (m_x*cos(roll)) + ...
%            m_y * sin(roll) * sin(pitch) + ...
%            m_z * cos(roll)  *sin(pitch));

== matlab function SensorFusionCompare/Quarternion EKF + Amfitrack (Yaw Only) - Simplified/MATLAB Function ==
  data: quat_in input; euler output
function euler = to_euler(quat_in)

q0 = quat_in(1);
q1 = quat_in(2);
q2 = quat_in(3);
q3 = quat_in(4);

roll = atan((2 * (q0*q1 + q2*q3))/(1 - 2*(q1^2 + q2^2)));
pitch = asin(2 * (q0*q2 - q1*q3));
yaw = atan2((2 * (q0*q3 + q1*q2)),(1 - 2*(q2^2 + q3^2)));

euler = [roll; pitch; yaw];

== matlab function SensorFusionCompare/Quarternion EKF + Amfitrack (Yaw Only) - Simplified/Predict ==
  data: quat_in input; q_t_dash output; omega input; delta_t input; P_t_dash output; P_t_ input; gyro_sigma input
function [q_t_dash, P_t_dash] = Predict(quat_in, omega, delta_t, P_t_, gyro_sigma)

q0 = quat_in(1);
q1 = quat_in(2);
q2 = quat_in(3);
q3 = quat_in(4);

omega_x = omega(1);
omega_y = omega(2);
omega_z = omega(3);

R_gyro = [gyro_sigma(1)^2 0 0;
          0 gyro_sigma(2)^2 0;
          0 0 gyro_sigma(3)^2;];

q0_out = q0 + delta_t/2 * (-omega_x * q1 - omega_y * q2 - omega_z * q3);
q1_out = q1 + delta_t/2 * ( omega_x * q0 - omega_y * q3 + omega_z * q2);
q2_out = q2 + delta_t/2 * ( omega_x * q3 + omega_y * q0 - omega_z * q1);
q3_out = q3 + delta_t/2 * (-omega_x * q2 + omega_y * q1 + omega_z * q0);

q_t_dash = quatnormalize([q0_out, q1_out, q2_out, q3_out]);

dt2 = delta_t/2;

F = [1  -dt2*omega_x -dt2*omega_y -dt2*omega_z;
    dt2*omega_x    1  dt2*omega_z  dt2*omega_y;
    dt2*omega_y   -dt2*omega_z   1 dt2*omega_x;
    dt2*omega_z    dt2*omega_y -dt2*omega_x  1;
    ];


W = dt2 * [-q1 -q2 -q3;
            q0 -q3  q2;
            q3  q0 -q1;
            -q2 q1  q0]; 

Q_t =  W* R_gyro * W';

P_t_dash = F * P_t_ * F' + Q_t;

== matlab function SensorFusionCompare/Quarternion EKF + Amfitrack (Yaw Only) - Simplified/Update ==
  data: accel input; q_meas input; q_t output; quat_in input; acc_sigma input; q_sigma input; P_t output; P_t_dash input; prev_yaw_mp input; prev_cul_yaw_mp input; yaw_mp output; yaw_cul_mp output
function [q_t, P_t, yaw_mp, yaw_cul_mp]   = Update(accel, q_meas, quat_in, acc_sigma, q_sigma, P_t_dash, prev_yaw_mp, prev_cul_yaw_mp)

%% Unbox function inputs
q0 = quat_in(1);
q1 = quat_in(2);
q2 = quat_in(3);
q3 = quat_in(4);

q_t_dash = [q0; q1; q2; q3];

yaw_meas_prev = prev_yaw_mp(1);
yaw_meas_cul_prev = prev_cul_yaw_mp(1);
yaw_pred_prev = prev_yaw_mp(2);
yaw_pred_cul_prev = prev_cul_yaw_mp(2);

yaw_meas = atan2((2 * (q_meas(1)*q_meas(4) + q_meas(2)*q_meas(3))),(1 - 2*(q_meas(3)^2 + q_meas(4)^2)));
yaw_pred = atan2((2 * (q0*q3 + q1*q2)),(1 - 2*(q2^2 + q3^2)));

%% Accumulate measured & predicted Yaw Angles
% Determine Change in measured and predicted Yaw angle
delta_yaw_meas = yaw_meas - yaw_meas_prev;
delta_yaw_pred = yaw_pred - yaw_pred_prev;

if delta_yaw_meas > pi
    delta_yaw_meas = delta_yaw_meas - 2*pi;
elseif delta_yaw_meas < -pi
    delta_yaw_meas = delta_yaw_meas + 2*pi;
end

yaw_meas_cul = yaw_meas_cul_prev + delta_yaw_meas;

if delta_yaw_pred > pi
    delta_yaw_pred = delta_yaw_pred - 2*pi;
elseif delta_yaw_pred < -pi
    delta_yaw_pred = delta_yaw_pred + 2*pi;
end

yaw_pred_cul = yaw_pred_cul_prev + delta_yaw_pred;

% Send them to the delay blocks for use in next update step
yaw_mp = [yaw_meas,yaw_pred];
yaw_cul_mp = [yaw_meas_cul, yaw_pred_cul];


%% Update State Estimation

% Construct measurement vector using accumulated yaw angles
z_t = [accel(1);
       accel(2);
       accel(3);
       yaw_meas_cul;
       ];

gx = 0;
gy = 0;
gz = 1;

R = [acc_sigma^2 * eye(3) zeros(3,1);
    zeros(1,3)     q_sigma^2 * eye(1)];

% Measurement Model
h = [
    2*(gx * (1/2 - q2^2 - q3^2) + gy * (q0*q3 + q1*q2) + gz * (q1*q3 - q0*q2));
    2*(gx * (q1*q2 - q0*q3) + gy * (1/2 - q1^2 - q3^2) + gz * (q0*q1 + q2*q3));
    2*(gx * (q0*q2 + q1*q3) + gy * (q2*q3 - q0*q1) + gz * (1/2 - q1^2 - q2^2));
                                    yaw_pred_cul                           ;
                                    
];

c_1 = 2*q2^2 + 2*q3^2 - 1;
c_2 = (2*q0*q3 + 2*q1*q2);
s = -2*(c_1^2 + c_2^2);
% Jacobian of Measurement Model
H = 2 * [
    gx*q0 + gy*q3 - gz*q2,  gx*q1 + gy*q2 + gz*q3, -gx*q2 + gy*q1 - gz*q0, -gx*q3 + gy*q0 + gz*q1;
   -gx*q3 + gy*q0 + gz*q1,  gx*q2 - gy*q1 + gz*q0,  gx*q1 + gy*q2 + gz*q3, -gx*q0 - gy*q3 + gz*q2;
    gx*q2 - gy*q1 + gz*q0,  gx*q3 - gy*q0 - gz*q1,  gx*q0 + gy*q3 - gz*q2,  gx*q1 + gy*q2 + gz*q3;
                                            
    (2*q3*(c_1))/s, (2*q2*(c_1))/s, ((2*q1)*c_1 - (4*q2*(c_2)))/s, (((2*q0)*c_1 - (4*q3*(c_2))))/s
];
%{
s = -((2*q3^2 - 1)^2 + (2*q0*q3)^2);
c = 2*q3^2 - 1;
H = 2 * [
    gx*q0 + gy*q3 - gz*q2,  gx*q1 + gy*q2 + gz*q3, -gx*q2 + gy*q1 - gz*q0, -gx*q3 + gy*q0 + gz*q1;
   -gx*q3 + gy*q0 + gz*q1,  gx*q2 - gy*q1 + gz*q0,  gx*q1 + gy*q2 + gz*q3, -gx*q0 - gy*q3 + gz*q2;
    gx*q2 - gy*q1 + gz*q0,  gx*q3 - gy*q0 - gz*q1,  gx*q0 + gy*q3 - gz*q2,  gx*q1 + gy*q2 + gz*q3;
                                            
    0.5*[(2*q3*(c))/s, (2*q2*(c))/s, (((2*q1)*c - (4*q2*(2*q0*q3))))/s, (((2*q0)*c - (4*q3*(2*q0*q3))))/s]
];
%}
v_t = z_t - h;

S_t = H * P_t_dash * transpose(H) + R;
K_t = P_t_dash * transpose(H) * inv(S_t);

q_t = quatnormalize(transpose(q_t_dash + K_t*v_t));

P_t = (eye(4) - K_t*H) * P_t_dash;

== matlab function SensorFusionCompare/Quarternion EKF + Amfitrack (Yaw Only) - Simplified/normalize_g_b ==
  data: v input; v_norm output
function v_norm = normalize_vec(v)

v_norm = v / norm(v);
